simulink model "ss_solver"  (R2021b)
settings: Solver=ode15s  StartTime=0.0  StopTime=5  RelTol=1e-5
undefined symbols (not defined in the file or in its folder): fss_fcn
settings Model: Creator=cosimodellasantina  LastModifiedBy=mrsub
settings SolverCC: AlgebraicLoopSolver=TrustRegion
settings DebuggingCC: SFMachineParentedDataDiag=warning
settings SFSimCC: CustomCodeUndefinedFunction=UseInterfaceOnly

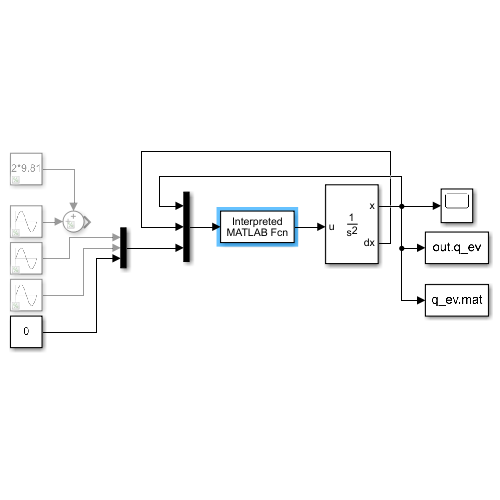
[thumbnail: Simulink's stored preview of the top-level diagram]
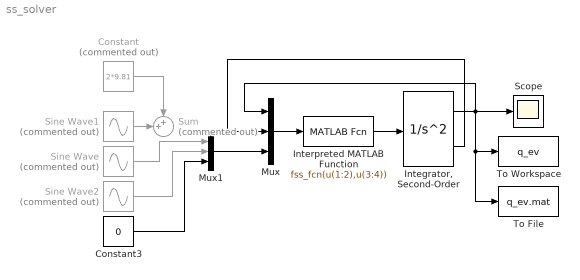
== system ss_solver ==
  Constant : Constant  Commented=on  Value=2*9.81
  Constant3 : Constant  Value=0
  "Integrator, Second-Order" : SecondOrderIntegrator  ICX=x_0  ICDXDT=dx_0
  Interpreted MATLAB Function : MATLABFcn  MATLABFcn=fss_fcn(u(1:2),u(3:4))
  Mux : Mux  Inputs=3
  Mux1 : Mux  Inputs=3
  Scope : Scope
  Sine Wave : Sin  Commented=on  Frequency=pi  SampleTime=0
  Sine Wave1 : Sin  Commented=on  Amplitude=0  Frequency=pi  SampleTime=0
  Sine Wave2 : Sin  Commented=on  Amplitude=2  Frequency=3*pi/2  SampleTime=0
  Sum : Sum  Commented=on  Inputs=++|
  To File : ToFile  Filename=q_ev.mat  SaveFormat=Timeseries
  To Workspace : ToWorkspace  VariableName=q_ev  SaveFormat=Timeseries  SampleTime=-1
  wires:
  Mux/1 -> Interpreted MATLAB Function/1
  Interpreted MATLAB Function/1 -> "Integrator, Second-Order"/1
  "Integrator, Second-Order"/1 -> Mux/1, To File/1, To Workspace/1, Scope/1
  Sine Wave1/1 -> Sum/2
  Constant/1 -> Sum/1
  Constant3/1 -> Mux1/3
  Mux1/1 -> Mux/3
  "Integrator, Second-Order"/2 -> Mux/2
  Sine Wave/1 -> Mux1/1
  Sine Wave2/1 -> Mux1/2
